simulink model "UAVFormation"  (R2021a)
settings: Solver=FixedStepAuto  StartTime=0.0  StopTime=150  FixedStep=0.1  RelTol=1e-3
(part 1 of 2)
settings Model: Creator=templ  LastModifiedBy=templ
settings DataIOCC: ReturnWorkspaceOutputs=off

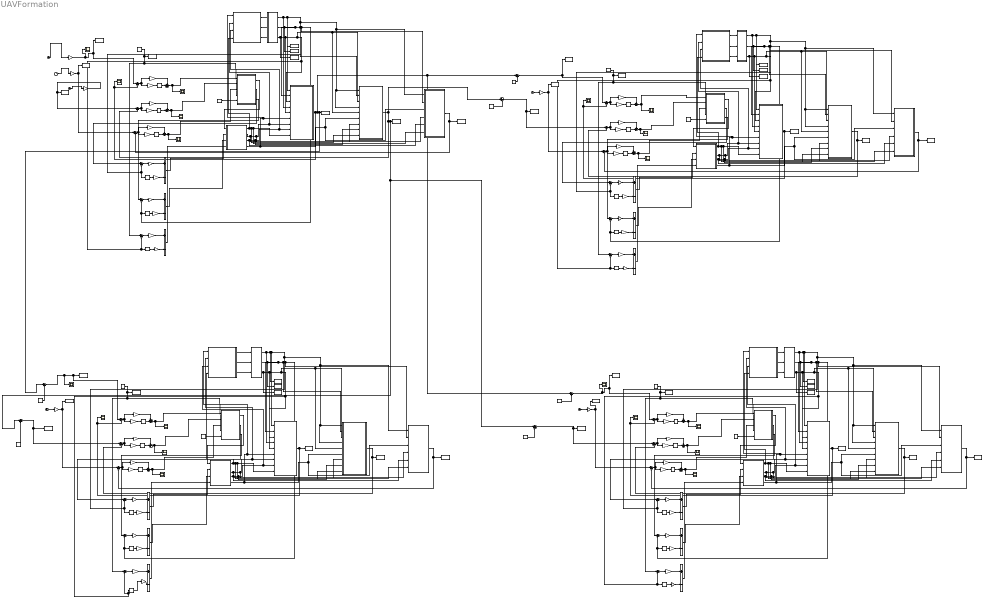
== system UAVFormation ==
  note: Attitude
  note: Position
  note: Attitude
  note: Position
  note: Attitude
  note: Position
  note: Attitude
  note: Position
  Add{1..12} (12 alike) : Sum  Inputs=+-
  Attitude Control Module1 : Subsystem
  Attitude Control Module2 : Subsystem
  Attitude Control Module3 : Subsystem
  Attitude Control Module4 : Subsystem
  Clock{,1,3,5,8,11} (6 alike) : Clock
  Constant{,1..5} (6 alike) : Constant  Value=5
  Derivative{1..24} (24 alike) : Derivative
  Gain{10,32,35,55} (4 alike) : Gain  Gain=0.05
  Gain{11,36,41,56} (4 alike) : Gain  Gain=0.32
  Gain{12..13,16,18,38,40,43,45,58,60} (10 alike) : Gain  Gain=0.2
  Gain{7,14,17,27,31,37,39,42,44,52,57,59} (12 alike) : Gain  Gain=0.5
  Gain{3,15,23,48} (4 alike) : Gain  Gain=0.1
  Gain{4,8,20,24,28,33,49,53} (8 alike) : Gain  Gain=0.6
  Gain{5,9,21,25,29,34,50,54} (8 alike) : Gain  Gain=0.8
  Gain{6,26,30,51} (4 alike) : Gain  Gain=0.25
  MATLAB Function1 : MATLAB Function  TreatAsAtomicUnit=on
  MATLAB Function2 : MATLAB Function  TreatAsAtomicUnit=on
  MATLAB Function3 : MATLAB Function  TreatAsAtomicUnit=on
  MATLAB Function4 : MATLAB Function  TreatAsAtomicUnit=on
  MATLAB Function5 : MATLAB Function  TreatAsAtomicUnit=on
  MATLAB Function6 : MATLAB Function  TreatAsAtomicUnit=on
  MATLAB Function7 : MATLAB Function  TreatAsAtomicUnit=on
  MATLAB Function8 : MATLAB Function  TreatAsAtomicUnit=on
  Position1 : MATLAB Function  TreatAsAtomicUnit=on
  Position2 : MATLAB Function  TreatAsAtomicUnit=on
  Position3 : MATLAB Function  TreatAsAtomicUnit=on
  Position4 : MATLAB Function  TreatAsAtomicUnit=on
  Scope{1..5,7..20} (19 alike) : Scope
  Subsystem1 : Subsystem
  Subsystem2 : Subsystem
  Subsystem3 : Subsystem
  Subsystem4 : Subsystem
  Subsystem5 : Subsystem
  Subsystem6 : Subsystem
  Subsystem7 : Subsystem
  Subsystem8 : Subsystem
  Sum{,2,4,6..9,11,13,15..18,21,23,25..28,30..31,33..38,41} (28 alike) : Sum  Inputs=|+-
  Sum{1,3,5,10,12,14,19..20,22,24,29,32} (12 alike) : Sum  Inputs=++|
  Sum39 : Sum  Inputs=|++
  Sum40 : Sum  Inputs=|++
  To Workspace1 : ToWorkspace  VariableName=theta1  SampleTime=-1
  To Workspace10 : ToWorkspace  VariableName=phi1  SampleTime=-1
  To Workspace11 : ToWorkspace  VariableName=xd1  SampleTime=-1
  To Workspace12 : ToWorkspace  VariableName=yd1  SampleTime=-1
  To Workspace13 : ToWorkspace  VariableName=zd1  SampleTime=-1
  To Workspace14 : ToWorkspace  VariableName=theta2  SampleTime=-1
  To Workspace15 : ToWorkspace  VariableName=psid2  SampleTime=-1
  To Workspace16 : ToWorkspace  VariableName=psi2  SampleTime=-1
  To Workspace17 : ToWorkspace  VariableName=x2  SampleTime=-1
  To Workspace18 : ToWorkspace  VariableName=y2  SampleTime=-1
  To Workspace19 : ToWorkspace  VariableName=z2  SampleTime=-1
  To Workspace2 : ToWorkspace  VariableName=psid1  SampleTime=-1
  To Workspace20 : ToWorkspace  VariableName=theta  SampleTime=-1
  To Workspace21 : ToWorkspace  VariableName=psid  SampleTime=-1
  To Workspace22 : ToWorkspace  VariableName=psi  SampleTime=-1
  To Workspace23 : ToWorkspace  VariableName=x  SampleTime=-1
  To Workspace24 : ToWorkspace  VariableName=y  SampleTime=-1
  To Workspace25 : ToWorkspace  VariableName=z  SampleTime=-1
  To Workspace26 : ToWorkspace  VariableName=phi2  SampleTime=-1
  To Workspace27 : ToWorkspace  VariableName=xd2  SampleTime=-1
  To Workspace28 : ToWorkspace  VariableName=yd2  SampleTime=-1
  To Workspace29 : ToWorkspace  VariableName=phi  SampleTime=-1
  To Workspace3 : ToWorkspace  VariableName=psi1  SampleTime=-1
  To Workspace30 : ToWorkspace  VariableName=zd2  SampleTime=-1
  To Workspace31 : ToWorkspace  VariableName=theta3  SampleTime=-1
  To Workspace32 : ToWorkspace  VariableName=psid3  SampleTime=-1
  To Workspace33 : ToWorkspace  VariableName=psi3  SampleTime=-1
  To Workspace34 : ToWorkspace  VariableName=x3  SampleTime=-1
  To Workspace35 : ToWorkspace  VariableName=y3  SampleTime=-1
  To Workspace36 : ToWorkspace  VariableName=z3  SampleTime=-1
  To Workspace37 : ToWorkspace  VariableName=phi3  SampleTime=-1
  To Workspace38 : ToWorkspace  VariableName=xd3  SampleTime=-1
  To Workspace39 : ToWorkspace  VariableName=yd3  SampleTime=-1
  To Workspace4 : ToWorkspace  VariableName=x1  SampleTime=-1
  To Workspace40 : ToWorkspace  VariableName=zd3  SampleTime=-1
  To Workspace5 : ToWorkspace  VariableName=y1  SampleTime=-1
  To Workspace6 : ToWorkspace  VariableName=xd  SampleTime=-1
  To Workspace7 : ToWorkspace  VariableName=yd  SampleTime=-1
  To Workspace8 : ToWorkspace  VariableName=zd  SampleTime=-1
  To Workspace9 : ToWorkspace  VariableName=z1  SampleTime=-1
  m{1..4} (4 alike) : Constant  Value=1.5
  psaid{1..4} (4 alike) : Constant  Value=0.2
  x1 : Subsystem
  x2 : Subsystem
  x3 : Subsystem
  x4 : Subsystem
  wires:
  MATLAB Function1/2(w2) -> Subsystem5/4(w2), Subsystem4/7(w2), Attitude Control Module2/2(w2), x2/7(w2)
  MATLAB Function1/3(w3) -> Subsystem5/5(w3), Subsystem4/8(w3), Attitude Control Module2/3(w3), x2/8(w3)
  MATLAB Function1/1(w1) -> Attitude Control Module2/4(w1), Subsystem4/9(w1), Subsystem5/6(w1), x2/9(w1)
  MATLAB Function1/4(w4) -> Subsystem5/3(w4), Subsystem4/6(w4), Attitude Control Module2/1(w4), x2/6(w4)
  Attitude Control Module2/1(phi) -> MATLAB Function5/1(u1)
  Attitude Control Module2/2(theta) -> MATLAB Function5/2(u2)
  Attitude Control Module2/3(psai) -> MATLAB Function5/3(u3)
  Gain20/1 -> Sum20/1
  Derivative16/1 -> Sum24/2
  Gain21/1 -> Derivative14/1
  Gain36/1 -> Derivative16/1
  Gain33/1 -> Sum22/1
  Sum30/1 -> Gain21/1, Gain20/1
  Derivative15/1 -> Sum22/2
  Sum21/1 -> Gain34/1, Gain33/1
  Subsystem5/1(Out1) -> Sum23/2, To Workspace25/1
  Gain35/1 -> Sum24/1
  Derivative14/1 -> Sum20/2
  Gain15/1 -> Sum23/1, To Workspace8/1
  Sum23/1 -> Gain36/1, Gain35/1
  Gain34/1 -> Derivative15/1
  Gain13/1 -> Sum21/1, To Workspace7/1
  Gain12/1 -> Scope3/1, To Workspace6/1, Sum30/1
  Position1/1(U1) -> MATLAB Function1/1(U1)
  Sum22/1 -> Scope12/1, Position1/2(Uy)
  Add8/1 -> MATLAB Function1/4(U4)
  m1/1 -> Position1/5(m)
  Add6/1 -> MATLAB Function1/2(U2)
  Sum24/1 -> Scope13/1, Position1/3(Uz)
  Add7/1 -> MATLAB Function1/3(U3)
  Sum20/1 -> Scope11/1, Position1/1(Ux)
  Sum27/1 -> Gain30/1
  Derivative13/1 -> Gain31/1
  Derivative17/1 -> Gain38/1
  Gain31/1 -> Add8/2
  Gain38/1 -> Add6/2
  Gain40/1 -> Add7/2
  MATLAB Function5/3(psai) -> To Workspace22/1, Subsystem4/5(In5), Subsystem4/3(psai), Sum27/2, Derivative13/1, x2/3(psai), x2/5(In5)
  Gain39/1 -> Add7/1
  Gain37/1 -> Add6/1
  Sum25/1 -> Gain37/1
  Position1/2(phid) -> Sum25/1
  Position1/3(thetad) -> Sum26/1
  Derivative12/1 -> Gain40/1
  psaid3/1 -> Sum27/1, Position1/4(psaid), To Workspace21/1
  Gain30/1 -> Add8/1
  MATLAB Function5/1(phi) -> x2/4(In4), To Workspace29/1, Derivative17/1, Sum25/2, Subsystem5/1(phi), Subsystem4/4(In4), Subsystem4/1(phi), x2/1(phi)
  MATLAB Function5/2(theta) -> To Workspace20/1, Sum26/2, Derivative12/1, Subsystem5/2(theta), Subsystem4/2(theta), x2/2(theta)
  Sum26/1 -> Gain39/1
  MATLAB Function2/4(w4) -> Subsystem2/3(w4), Subsystem1/6(w4), Attitude Control Module1/1(w4), x1/6(w4)
  Add1/1 -> MATLAB Function2/2(U2)
  Sum7/1 -> Gain17/1
  Sum37/1 -> Sum2/1, To Workspace12/1
  Clock5/1 -> Gain3/1
  Sum/1 -> To Workspace11/1, Sum9/1
  Gain6/1 -> Add3/1
  Sum6/1 -> Gain14/1
  Derivative1/1 -> Gain18/1
  Gain17/1 -> Add2/1
  Gain18/1 -> Add2/2
  Add2/1 -> MATLAB Function2/3(U3)
  Gain14/1 -> Add1/1
  Add3/1 -> MATLAB Function2/4(U4)
  Gain16/1 -> Add1/2
  Derivative2/1 -> Gain7/1
  Sum8/1 -> Gain6/1
  Derivative6/1 -> Gain16/1
  Gain3/1 -> Sum4/1, To Workspace13/1
  MATLAB Function2/1(w1) -> Attitude Control Module1/4(w1), Subsystem1/9(w1), Subsystem2/6(w1), x1/9(w1)
  m2/1 -> Position2/5(m)
  MATLAB Function2/3(w3) -> Subsystem2/5(w3), Subsystem1/8(w3), Attitude Control Module1/3(w3), x1/8(w3)
  Subsystem2/1(Out1) -> Sum4/2, To Workspace9/1
  x1/1(Out1) -> Sum9/2, Scope5/1, To Workspace4/1
  Gain9/1 -> Derivative4/1
  Sum1/1 -> Scope1/1, Position2/1(Ux)
  Position2/1(U1) -> MATLAB Function2/1(U1)
  Position2/2(phid) -> Sum6/1
  Gain4/1 -> Sum1/1
  Gain7/1 -> Add3/2
  Gain10/1 -> Sum5/1
  Sum2/1 -> Gain9/1, Gain8/1
  Derivative3/1 -> Sum1/2
  MATLAB Function2/2(w2) -> Subsystem2/4(w2), Subsystem1/7(w2), Attitude Control Module1/2(w2), x1/7(w2)
  MATLAB Function3/1(phi) -> x1/4(In4), To Workspace10/1, Derivative6/1, Sum6/2, Subsystem2/1(phi), Subsystem1/4(In4), Subsystem1/1(phi), x1/1(phi)
  Attitude Control Module1/3(psai) -> MATLAB Function3/3(u3)
  Sum5/1 -> Scope4/1, Position2/3(Uz)
  Position2/3(thetad) -> Sum7/1
  Sum4/1 -> Gain11/1, Gain10/1
  Gain8/1 -> Sum3/1
  Sum9/1 -> Gain5/1, Gain4/1
  Gain11/1 -> Derivative5/1
  Derivative5/1 -> Sum5/2
  Derivative4/1 -> Sum3/2
  Subsystem1/1(Out1) -> Sum2/2, To Workspace5/1
  Gain5/1 -> Derivative3/1
  Attitude Control Module1/2(theta) -> MATLAB Function3/2(u2)
  MATLAB Function3/3(psai) -> To Workspace3/1, Subsystem1/5(In5), Subsystem1/3(psai), Sum8/2, Derivative2/1, x1/3(psai), x1/5(In5)
  Sum3/1 -> Scope2/1, Position2/2(Uy)
  MATLAB Function3/2(theta) -> To Workspace1/1, Sum7/2, Derivative1/1, Subsystem2/2(theta), Subsystem1/2(theta), x1/2(theta)
  psaid1/1 -> Sum8/1, Position2/4(psaid), To Workspace2/1
  Attitude Control Module1/1(phi) -> MATLAB Function3/1(u1)
  MATLAB Function4/4(w4) -> Subsystem6/3(w4), Subsystem3/6(w4), Attitude Control Module3/1(w4), x3/6(w4)
  Add4/1 -> MATLAB Function4/2(U2)
  Sum16/1 -> Gain44/1
  Clock8/1 -> Gain23/1
  Gain26/1 -> Add9/1
  Sum15/1 -> Gain42/1
  Derivative7/1 -> Gain45/1
  Gain44/1 -> Add5/1
  Gain45/1 -> Add5/2
  Add5/1 -> MATLAB Function4/3(U3)
  Gain42/1 -> Add4/1
  Add9/1 -> MATLAB Function4/4(U4)
  Gain43/1 -> Add4/2
  Derivative8/1 -> Gain27/1
  Sum17/1 -> Gain26/1
  Derivative18/1 -> Gain43/1
  Gain23/1 -> Sum13/1, To Workspace30/1
  MATLAB Function4/1(w1) -> Attitude Control Module3/4(w1), Subsystem3/9(w1), Subsystem6/6(w1), x3/9(w1)
  m3/1 -> Position3/5(m)
  MATLAB Function4/3(w3) -> Subsystem6/5(w3), Subsystem3/8(w3), Attitude Control Module3/3(w3), x3/8(w3)
  Subsystem6/1(Out1) -> Sum13/2, To Workspace19/1
  x3/1(Out1) -> Sum18/2, Scope10/1, To Workspace17/1
  Gain29/1 -> Derivative10/1
  Sum10/1 -> Scope7/1, Position3/1(Ux)
  Position3/1(U1) -> MATLAB Function4/1(U1)
  Position3/2(phid) -> Sum15/1
  Gain24/1 -> Sum10/1
  Gain27/1 -> Add9/2
  Gain32/1 -> Sum14/1
  Sum11/1 -> Gain29/1, Gain28/1
  Derivative9/1 -> Sum10/2
  MATLAB Function4/2(w2) -> Subsystem6/4(w2), Subsystem3/7(w2), Attitude Control Module3/2(w2), x3/7(w2)
  MATLAB Function6/1(phi) -> x3/4(In4), To Workspace26/1, Derivative18/1, Sum15/2, Subsystem6/1(phi), Subsystem3/4(In4), Subsystem3/1(phi), x3/1(phi)
  Attitude Control Module3/3(psai) -> MATLAB Function6/3(u3)
  Sum14/1 -> Scope9/1, Position3/3(Uz)
  Position3/3(thetad) -> Sum16/1
  Sum13/1 -> Gain41/1, Gain32/1
  Gain28/1 -> Sum12/1
  Sum18/1 -> Gain25/1, Gain24/1
  Gain41/1 -> Derivative11/1
  Derivative11/1 -> Sum14/2
  Derivative10/1 -> Sum12/2
  Subsystem3/1(Out1) -> Sum11/2, To Workspace18/1
  Gain25/1 -> Derivative9/1
  Attitude Control Module3/2(theta) -> MATLAB Function6/2(u2)
  MATLAB Function6/3(psai) -> To Workspace16/1, Subsystem3/5(In5), Subsystem3/3(psai), Derivative8/1, Sum17/2, x3/3(psai), x3/5(In5)
  Sum12/1 -> Scope8/1, Position3/2(Uy)
  MATLAB Function6/2(theta) -> To Workspace14/1, Sum16/2, Derivative7/1, Subsystem6/2(theta), Subsystem3/2(theta), x3/2(theta)
  psaid2/1 -> Sum17/1, Position3/4(psaid), To Workspace15/1
  Attitude Control Module3/1(phi) -> MATLAB Function6/1(u1)
  MATLAB Function7/4(w4) -> Subsystem8/3(w4), Subsystem7/6(w4), Attitude Control Module4/1(w4), x4/6(w4)
  Add10/1 -> MATLAB Function7/2(U2)
  Sum34/1 -> Gain59/1
  Sum41/1 -> Sum28/1, To Workspace39/1
  Clock11/1 -> Gain48/1
  Sum40/1 -> Scope20/1, To Workspace38/1, Sum36/1
  Gain51/1 -> Add12/1
  Sum33/1 -> Gain57/1
  Derivative19/1 -> Gain60/1
  Gain59/1 -> Add11/1
  Gain60/1 -> Add11/2
  Add11/1 -> MATLAB Function7/3(U3)
  Gain57/1 -> Add10/1
  Add12/1 -> MATLAB Function7/4(U4)
  Gain58/1 -> Add10/2
  Derivative20/1 -> Gain52/1
  Sum35/1 -> Gain51/1
  Derivative24/1 -> Gain58/1
  Gain48/1 -> Sum31/1, To Workspace40/1
  MATLAB Function7/1(w1) -> Attitude Control Module4/4(w1), Subsystem7/9(w1), Subsystem8/6(w1), x4/9(w1)
  m4/1 -> Position4/5(m)
  MATLAB Function7/3(w3) -> Subsystem8/5(w3), Subsystem7/8(w3), Attitude Control Module4/3(w3), x4/8(w3)
  Subsystem8/1(Out1) -> Sum31/2, To Workspace36/1
  x4/1(Out1) -> Sum36/2, Scope19/1, To Workspace34/1
  Gain54/1 -> Derivative22/1
  Sum19/1 -> Scope16/1, Position4/1(Ux)
  Position4/1(U1) -> MATLAB Function7/1(U1)
  Position4/2(phid) -> Sum33/1
  Gain49/1 -> Sum19/1
  Gain52/1 -> Add12/2
  Gain55/1 -> Sum32/1
  Sum28/1 -> Gain54/1, Gain53/1
  Derivative21/1 -> Sum19/2
  MATLAB Function7/2(w2) -> Subsystem8/4(w2), Subsystem7/7(w2), Attitude Control Module4/2(w2), x4/7(w2)
  MATLAB Function8/1(phi) -> x4/4(In4), To Workspace37/1, Derivative24/1, Sum33/2, Subsystem8/1(phi), Subsystem7/4(In4), Subsystem7/1(phi), x4/1(phi)
  Attitude Control Module4/3(psai) -> MATLAB Function8/3(u3)
  Sum32/1 -> Scope18/1, Position4/3(Uz)
  Position4/3(thetad) -> Sum34/1
  Sum31/1 -> Gain56/1, Gain55/1
  Gain53/1 -> Sum29/1
  Sum36/1 -> Gain50/1, Gain49/1
  Gain56/1 -> Derivative23/1
  Derivative23/1 -> Sum32/2
  Derivative22/1 -> Sum29/2
  Subsystem7/1(Out1) -> Sum28/2, To Workspace35/1
  Gain50/1 -> Derivative21/1
  Attitude Control Module4/2(theta) -> MATLAB Function8/2(u2)
  MATLAB Function8/3(psai) -> To Workspace33/1, Subsystem7/5(In5), Subsystem7/3(psai), Sum35/2, Derivative20/1, x4/3(psai), x4/5(In5)
  Sum29/1 -> Scope17/1, Position4/2(Uy)
  MATLAB Function8/2(theta) -> To Workspace31/1, Sum34/2, Derivative19/1, Subsystem8/2(theta), Subsystem7/2(theta), x4/2(theta)
  psaid4/1 -> Sum35/1, Position4/4(psaid), To Workspace32/1
  Attitude Control Module4/1(phi) -> MATLAB Function8/1(u1)
  Constant/1 -> Sum/2
  Constant1/1 -> Sum37/2
  Constant2/1 -> Sum38/2
  Sum38/1 -> Scope15/1, Sum18/1, To Workspace27/1
  Sum39/1 -> Sum11/1, To Workspace28/1
  Constant3/1 -> Sum39/2
  Constant4/1 -> Sum40/2
  Constant5/1 -> Sum41/2
  x2/1(Out1) -> Sum30/2, Scope14/1, Sum40/1, Sum/1, Sum38/1, To Workspace23/1
  Subsystem4/1(Out1) -> Sum21/2, To Workspace24/1, Sum41/1, Sum39/1, Sum37/1
  Clock3/1 -> Gain15/1
  Clock/1 -> Gain12/1
  Clock1/1 -> Gain13/1

== system UAVFormation/Attitude Control Module1 ==
  note: phi
  note: theta
  note: psi
  w4 : Inport
  w2 : Inport  Port=2
  w3 : Inport  Port=3
  w1 : Inport  Port=4
  Integrator{,1..5} (6 alike) : Integrator
  Subsystem : Subsystem
  Subsystem1 : Subsystem
  Subsystem2 : Subsystem
  phi : Outport  VectorParamsAs1DForOutWhenUnconnected=off
  theta : Outport  Port=2  VectorParamsAs1DForOutWhenUnconnected=off
  psai : Outport  Port=3  VectorParamsAs1DForOutWhenUnconnected=off
  wires:
  w2/1 -> Subsystem2/2(w2), Subsystem/1(w2)
  Subsystem/1(Out1) -> Integrator1/1
  Integrator3/1 -> Subsystem2/4(In4), Subsystem/3(In3), Integrator2/1
  Integrator1/1 -> Subsystem2/3(In3), Subsystem1/3(In3), Integrator/1
  Integrator5/1 -> Subsystem/4(In4), Subsystem1/4(In4), Integrator4/1
  w4/1 -> Subsystem2/6(w4), Subsystem/2(w4)
  Subsystem2/1(Out1) -> Integrator5/1
  w1/1 -> Subsystem2/1(w1), Subsystem1/2(w1)
  Integrator2/1 -> theta/1
  Integrator/1 -> phi/1
  Integrator4/1 -> psai/1
  Subsystem1/1(Out1) -> Integrator3/1
  w3/1 -> Subsystem2/5(w3), Subsystem1/1(w3)

== system UAVFormation/Attitude Control Module2 ==
  note: phi
  note: theta
  note: psi
  w4 : Inport
  w2 : Inport  Port=2
  w3 : Inport  Port=3
  w1 : Inport  Port=4
  Integrator{,1..5} (6 alike) : Integrator
  Subsystem : Subsystem
  Subsystem1 : Subsystem
  Subsystem2 : Subsystem
  phi : Outport  VectorParamsAs1DForOutWhenUnconnected=off
  theta : Outport  Port=2  VectorParamsAs1DForOutWhenUnconnected=off
  psai : Outport  Port=3  VectorParamsAs1DForOutWhenUnconnected=off
  wires:
  w2/1 -> Subsystem2/2(w2), Subsystem/1(w2)
  Subsystem/1(Out1) -> Integrator1/1
  Integrator3/1 -> Subsystem2/4(In4), Subsystem/3(In3), Integrator2/1
  Integrator1/1 -> Subsystem2/3(In3), Subsystem1/3(In3), Integrator/1
  Integrator5/1 -> Subsystem/4(In4), Subsystem1/4(In4), Integrator4/1
  w4/1 -> Subsystem2/6(w4), Subsystem/2(w4)
  Subsystem2/1(Out1) -> Integrator5/1
  w1/1 -> Subsystem2/1(w1), Subsystem1/2(w1)
  Integrator2/1 -> theta/1
  Integrator/1 -> phi/1
  Integrator4/1 -> psai/1
  Subsystem1/1(Out1) -> Integrator3/1
  w3/1 -> Subsystem2/5(w3), Subsystem1/1(w3)

== system UAVFormation/Attitude Control Module3 ==
  note: phi
  note: theta
  note: psi
  w4 : Inport
  w2 : Inport  Port=2
  w3 : Inport  Port=3
  w1 : Inport  Port=4
  Integrator{,1..5} (6 alike) : Integrator
  Subsystem : Subsystem
  Subsystem1 : Subsystem
  Subsystem2 : Subsystem
  phi : Outport  VectorParamsAs1DForOutWhenUnconnected=off
  theta : Outport  Port=2  VectorParamsAs1DForOutWhenUnconnected=off
  psai : Outport  Port=3  VectorParamsAs1DForOutWhenUnconnected=off
  wires:
  w2/1 -> Subsystem2/2(w2), Subsystem/1(w2)
  Subsystem/1(Out1) -> Integrator1/1
  Integrator3/1 -> Subsystem2/4(In4), Subsystem/3(In3), Integrator2/1
  Integrator1/1 -> Subsystem2/3(In3), Subsystem1/3(In3), Integrator/1
  Integrator5/1 -> Subsystem/4(In4), Subsystem1/4(In4), Integrator4/1
  w4/1 -> Subsystem2/6(w4), Subsystem/2(w4)
  Subsystem2/1(Out1) -> Integrator5/1
  w1/1 -> Subsystem2/1(w1), Subsystem1/2(w1)
  Integrator2/1 -> theta/1
  Integrator/1 -> phi/1
  Integrator4/1 -> psai/1
  Subsystem1/1(Out1) -> Integrator3/1
  w3/1 -> Subsystem2/5(w3), Subsystem1/1(w3)

== system UAVFormation/Attitude Control Module4 ==
  note: phi
  note: theta
  note: psi
  w4 : Inport
  w2 : Inport  Port=2
  w3 : Inport  Port=3
  w1 : Inport  Port=4
  Integrator{,1..5} (6 alike) : Integrator
  Subsystem : Subsystem
  Subsystem1 : Subsystem
  Subsystem2 : Subsystem
  phi : Outport  VectorParamsAs1DForOutWhenUnconnected=off
  theta : Outport  Port=2  VectorParamsAs1DForOutWhenUnconnected=off
  psai : Outport  Port=3  VectorParamsAs1DForOutWhenUnconnected=off
  wires:
  w2/1 -> Subsystem2/2(w2), Subsystem/1(w2)
  Subsystem/1(Out1) -> Integrator1/1
  Integrator3/1 -> Subsystem2/4(In4), Subsystem/3(In3), Integrator2/1
  Integrator1/1 -> Subsystem2/3(In3), Subsystem1/3(In3), Integrator/1
  Integrator5/1 -> Subsystem/4(In4), Subsystem1/4(In4), Integrator4/1
  w4/1 -> Subsystem2/6(w4), Subsystem/2(w4)
  Subsystem2/1(Out1) -> Integrator5/1
  w1/1 -> Subsystem2/1(w1), Subsystem1/2(w1)
  Integrator2/1 -> theta/1
  Integrator/1 -> phi/1
  Integrator4/1 -> psai/1
  Subsystem1/1(Out1) -> Integrator3/1
  w3/1 -> Subsystem2/5(w3), Subsystem1/1(w3)

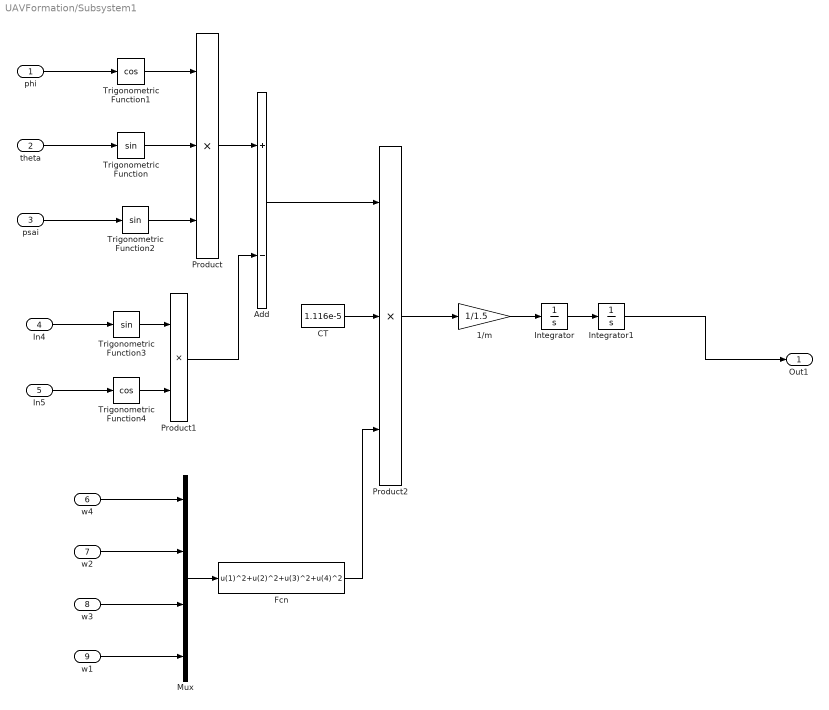
== system UAVFormation/Subsystem1 ==
  phi : Inport
  theta : Inport  Port=2
  psai : Inport  Port=3
  In4 : Inport  Port=4
  In5 : Inport  Port=5
  w4 : Inport  Port=6
  w2 : Inport  Port=7
  w3 : Inport  Port=8
  w1 : Inport  Port=9
  1/m : Gain  Gain=1/1.5
  Add : Sum  Inputs=+-
  CT : Constant  Value=1.116e-5
  Fcn : Fcn  Expr=u(1)^2+u(2)^2+u(3)^2+u(4)^2
  Integrator : Integrator
  Integrator1 : Integrator
  Mux : Mux
  Product : Product  Inputs=3
  Product1 : Product
  Product2 : Product  Inputs=3
  Trigonometric Function : Trigonometry
  Trigonometric Function1 : Trigonometry  Operator=cos
  Trigonometric Function2 : Trigonometry
  Trigonometric Function3 : Trigonometry
  Trigonometric Function4 : Trigonometry  Operator=cos
  Out1 : Outport  VectorParamsAs1DForOutWhenUnconnected=off
  wires:
  Mux/1 -> Fcn/1
  Product2/1 -> 1/m/1
  Fcn/1 -> Product2/3
  CT/1 -> Product2/2
  Trigonometric Function2/1 -> Product/3
  Trigonometric Function/1 -> Product/2
  Trigonometric Function3/1 -> Product1/1
  Product1/1 -> Add/2
  Product/1 -> Add/1
  Add/1 -> Product2/1
  In4/1 -> Trigonometric Function3/1
  Trigonometric Function1/1 -> Product/1
  Integrator/1 -> Integrator1/1
  w3/1 -> Mux/3
  Trigonometric Function4/1 -> Product1/2
  1/m/1 -> Integrator/1
  Integrator1/1 -> Out1/1
  w1/1 -> Mux/4
  phi/1 -> Trigonometric Function1/1
  w4/1 -> Mux/1
  In5/1 -> Trigonometric Function4/1
  w2/1 -> Mux/2
  psai/1 -> Trigonometric Function2/1
  theta/1 -> Trigonometric Function/1

== system UAVFormation/Subsystem2 ==
  phi : Inport
  theta : Inport  Port=2
  w4 : Inport  Port=3
  w2 : Inport  Port=4
  w3 : Inport  Port=5
  w1 : Inport  Port=6
  1/m : Gain  Gain=1/1.5
  Add : Sum  Inputs=+-
  CT : Constant  Value=1.116e-5
  Fcn : Fcn  Expr=u(1)^2+u(2)^2+u(3)^2+u(4)^2
  Integrator : Integrator
  Integrator1 : Integrator
  Mux : Mux
  Product1 : Product  Inputs=4
  Trigonometric Function : Trigonometry  Operator=cos
  Trigonometric Function1 : Trigonometry  Operator=cos
  mg : Constant  Value=1.5*9.81
  Out1 : Outport  VectorParamsAs1DForOutWhenUnconnected=off
  wires:
  Trigonometric Function1/1 -> Product1/1
  Integrator/1 -> Integrator1/1
  Fcn/1 -> Product1/4
  mg/1 -> Add/2
  CT/1 -> Product1/3
  Add/1 -> 1/m/1
  Mux/1 -> Fcn/1
  theta/1 -> Trigonometric Function/1
  1/m/1 -> Integrator/1
  Trigonometric Function/1 -> Product1/2
  Product1/1 -> Add/1
  w2/1 -> Mux/2
  Integrator1/1 -> Out1/1
  w3/1 -> Mux/3
  w4/1 -> Mux/1
  w1/1 -> Mux/4
  phi/1 -> Trigonometric Function1/1

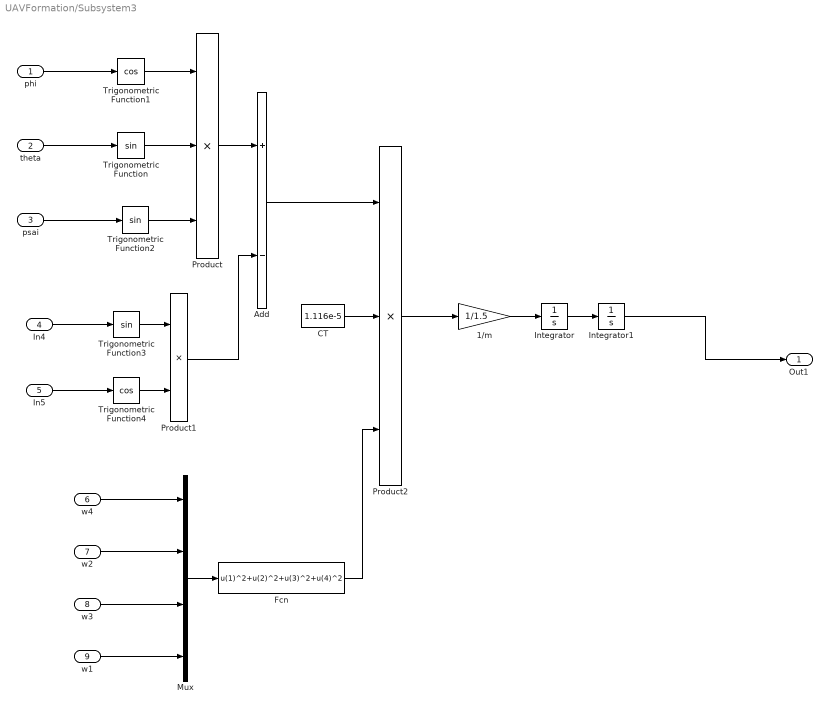
== system UAVFormation/Subsystem3 ==
  phi : Inport
  theta : Inport  Port=2
  psai : Inport  Port=3
  In4 : Inport  Port=4
  In5 : Inport  Port=5
  w4 : Inport  Port=6
  w2 : Inport  Port=7
  w3 : Inport  Port=8
  w1 : Inport  Port=9
  1/m : Gain  Gain=1/1.5
  Add : Sum  Inputs=+-
  CT : Constant  Value=1.116e-5
  Fcn : Fcn  Expr=u(1)^2+u(2)^2+u(3)^2+u(4)^2
  Integrator : Integrator
  Integrator1 : Integrator
  Mux : Mux
  Product : Product  Inputs=3
  Product1 : Product
  Product2 : Product  Inputs=3
  Trigonometric Function : Trigonometry
  Trigonometric Function1 : Trigonometry  Operator=cos
  Trigonometric Function2 : Trigonometry
  Trigonometric Function3 : Trigonometry
  Trigonometric Function4 : Trigonometry  Operator=cos
  Out1 : Outport  VectorParamsAs1DForOutWhenUnconnected=off
  wires:
  Mux/1 -> Fcn/1
  Product2/1 -> 1/m/1
  Fcn/1 -> Product2/3
  CT/1 -> Product2/2
  Trigonometric Function2/1 -> Product/3
  Trigonometric Function/1 -> Product/2
  Trigonometric Function3/1 -> Product1/1
  Product1/1 -> Add/2
  Product/1 -> Add/1
  Add/1 -> Product2/1
  In4/1 -> Trigonometric Function3/1
  Trigonometric Function1/1 -> Product/1
  Integrator/1 -> Integrator1/1
  w3/1 -> Mux/3
  Trigonometric Function4/1 -> Product1/2
  1/m/1 -> Integrator/1
  Integrator1/1 -> Out1/1
  w1/1 -> Mux/4
  phi/1 -> Trigonometric Function1/1
  w4/1 -> Mux/1
  In5/1 -> Trigonometric Function4/1
  w2/1 -> Mux/2
  psai/1 -> Trigonometric Function2/1
  theta/1 -> Trigonometric Function/1

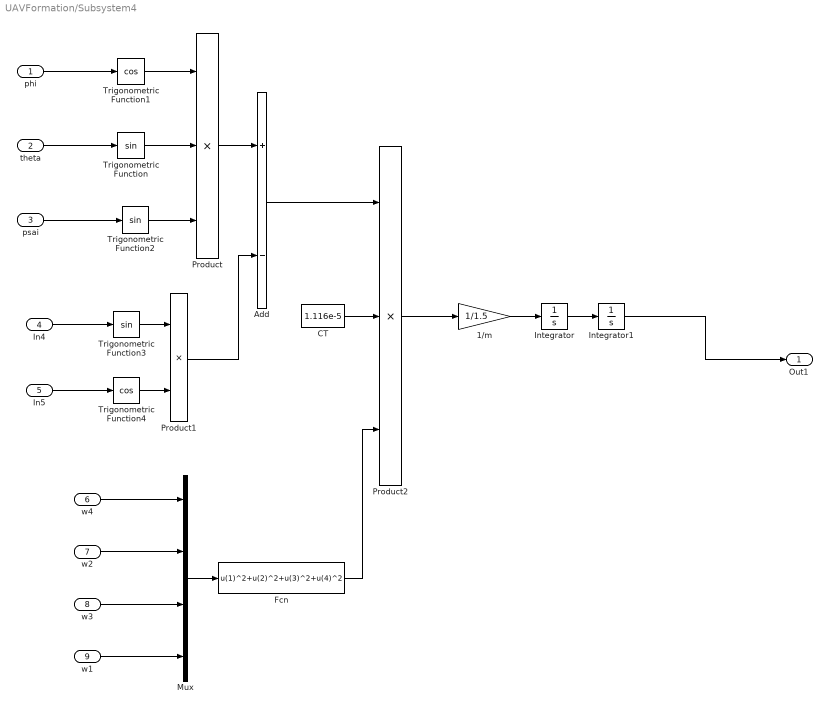
== system UAVFormation/Subsystem4 ==
  phi : Inport
  theta : Inport  Port=2
  psai : Inport  Port=3
  In4 : Inport  Port=4
  In5 : Inport  Port=5
  w4 : Inport  Port=6
  w2 : Inport  Port=7
  w3 : Inport  Port=8
  w1 : Inport  Port=9
  1/m : Gain  Gain=1/1.5
  Add : Sum  Inputs=+-
  CT : Constant  Value=1.116e-5
  Fcn : Fcn  Expr=u(1)^2+u(2)^2+u(3)^2+u(4)^2
  Integrator : Integrator
  Integrator1 : Integrator
  Mux : Mux
  Product : Product  Inputs=3
  Product1 : Product
  Product2 : Product  Inputs=3
  Trigonometric Function : Trigonometry
  Trigonometric Function1 : Trigonometry  Operator=cos
  Trigonometric Function2 : Trigonometry
  Trigonometric Function3 : Trigonometry
  Trigonometric Function4 : Trigonometry  Operator=cos
  Out1 : Outport  VectorParamsAs1DForOutWhenUnconnected=off
  wires:
  Mux/1 -> Fcn/1
  Product2/1 -> 1/m/1
  Fcn/1 -> Product2/3
  CT/1 -> Product2/2
  Trigonometric Function2/1 -> Product/3
  Trigonometric Function/1 -> Product/2
  Trigonometric Function3/1 -> Product1/1
  Product1/1 -> Add/2
  Product/1 -> Add/1
  Add/1 -> Product2/1
  In4/1 -> Trigonometric Function3/1
  Trigonometric Function1/1 -> Product/1
  Integrator/1 -> Integrator1/1
  w3/1 -> Mux/3
  Trigonometric Function4/1 -> Product1/2
  1/m/1 -> Integrator/1
  Integrator1/1 -> Out1/1
  w1/1 -> Mux/4
  phi/1 -> Trigonometric Function1/1
  w4/1 -> Mux/1
  In5/1 -> Trigonometric Function4/1
  w2/1 -> Mux/2
  psai/1 -> Trigonometric Function2/1
  theta/1 -> Trigonometric Function/1

== system UAVFormation/Subsystem5 ==
  phi : Inport
  theta : Inport  Port=2
  w4 : Inport  Port=3
  w2 : Inport  Port=4
  w3 : Inport  Port=5
  w1 : Inport  Port=6
  1/m : Gain  Gain=1/1.5
  Add : Sum  Inputs=+-
  CT : Constant  Value=1.116e-5
  Fcn : Fcn  Expr=u(1)^2+u(2)^2+u(3)^2+u(4)^2
  Integrator : Integrator
  Integrator1 : Integrator
  Mux : Mux
  Product1 : Product  Inputs=4
  Trigonometric Function : Trigonometry  Operator=cos
  Trigonometric Function1 : Trigonometry  Operator=cos
  mg : Constant  Value=1.5*9.81
  Out1 : Outport  VectorParamsAs1DForOutWhenUnconnected=off
  wires:
  Trigonometric Function1/1 -> Product1/1
  Integrator/1 -> Integrator1/1
  Fcn/1 -> Product1/4
  mg/1 -> Add/2
  CT/1 -> Product1/3
  Add/1 -> 1/m/1
  Mux/1 -> Fcn/1
  theta/1 -> Trigonometric Function/1
  1/m/1 -> Integrator/1
  Trigonometric Function/1 -> Product1/2
  Product1/1 -> Add/1
  w2/1 -> Mux/2
  Integrator1/1 -> Out1/1
  w3/1 -> Mux/3
  w4/1 -> Mux/1
  w1/1 -> Mux/4
  phi/1 -> Trigonometric Function1/1

== system UAVFormation/Subsystem6 ==
  phi : Inport
  theta : Inport  Port=2
  w4 : Inport  Port=3
  w2 : Inport  Port=4
  w3 : Inport  Port=5
  w1 : Inport  Port=6
  1/m : Gain  Gain=1/1.5
  Add : Sum  Inputs=+-
  CT : Constant  Value=1.116e-5
  Fcn : Fcn  Expr=u(1)^2+u(2)^2+u(3)^2+u(4)^2
  Integrator : Integrator
  Integrator1 : Integrator
  Mux : Mux
  Product1 : Product  Inputs=4
  Trigonometric Function : Trigonometry  Operator=cos
  Trigonometric Function1 : Trigonometry  Operator=cos
  mg : Constant  Value=1.5*9.81
  Out1 : Outport  VectorParamsAs1DForOutWhenUnconnected=off
  wires:
  Trigonometric Function1/1 -> Product1/1
  Integrator/1 -> Integrator1/1
  Fcn/1 -> Product1/4
  mg/1 -> Add/2
  CT/1 -> Product1/3
  Add/1 -> 1/m/1
  Mux/1 -> Fcn/1
  theta/1 -> Trigonometric Function/1
  1/m/1 -> Integrator/1
  Trigonometric Function/1 -> Product1/2
  Product1/1 -> Add/1
  w2/1 -> Mux/2
  Integrator1/1 -> Out1/1
  w3/1 -> Mux/3
  w4/1 -> Mux/1
  w1/1 -> Mux/4
  phi/1 -> Trigonometric Function1/1

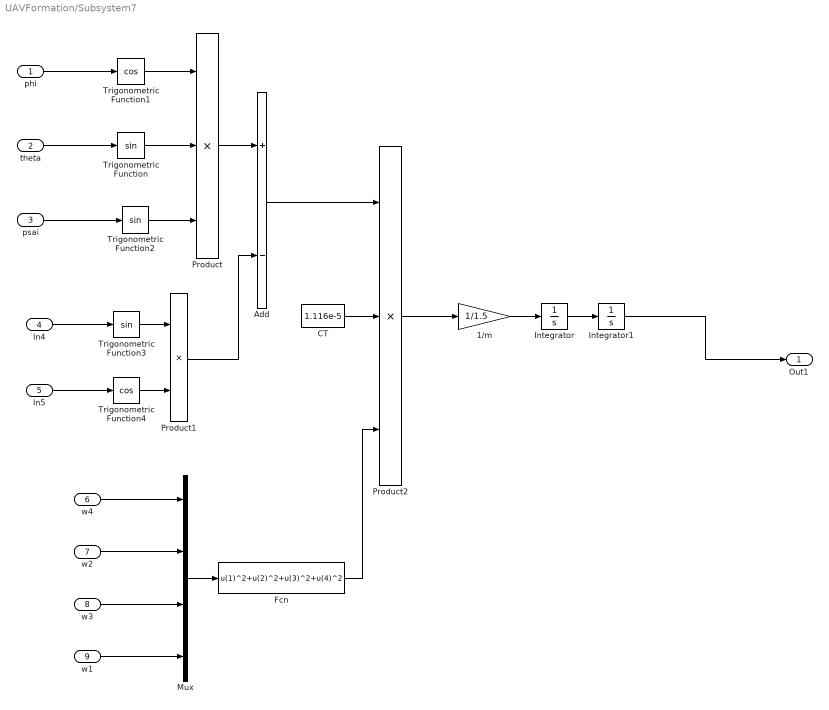
== system UAVFormation/Subsystem7 ==
  phi : Inport
  theta : Inport  Port=2
  psai : Inport  Port=3
  In4 : Inport  Port=4
  In5 : Inport  Port=5
  w4 : Inport  Port=6
  w2 : Inport  Port=7
  w3 : Inport  Port=8
  w1 : Inport  Port=9
  1/m : Gain  Gain=1/1.5
  Add : Sum  Inputs=+-
  CT : Constant  Value=1.116e-5
  Fcn : Fcn  Expr=u(1)^2+u(2)^2+u(3)^2+u(4)^2
  Integrator : Integrator
  Integrator1 : Integrator
  Mux : Mux
  Product : Product  Inputs=3
  Product1 : Product
  Product2 : Product  Inputs=3
  Trigonometric Function : Trigonometry
  Trigonometric Function1 : Trigonometry  Operator=cos
  Trigonometric Function2 : Trigonometry
  Trigonometric Function3 : Trigonometry
  Trigonometric Function4 : Trigonometry  Operator=cos
  Out1 : Outport  VectorParamsAs1DForOutWhenUnconnected=off
  wires:
  Mux/1 -> Fcn/1
  Product2/1 -> 1/m/1
  Fcn/1 -> Product2/3
  CT/1 -> Product2/2
  Trigonometric Function2/1 -> Product/3
  Trigonometric Function/1 -> Product/2
  Trigonometric Function3/1 -> Product1/1
  Product1/1 -> Add/2
  Product/1 -> Add/1
  Add/1 -> Product2/1
  In4/1 -> Trigonometric Function3/1
  Trigonometric Function1/1 -> Product/1
  Integrator/1 -> Integrator1/1
  w3/1 -> Mux/3
  Trigonometric Function4/1 -> Product1/2
  1/m/1 -> Integrator/1
  Integrator1/1 -> Out1/1
  w1/1 -> Mux/4
  phi/1 -> Trigonometric Function1/1
  w4/1 -> Mux/1
  In5/1 -> Trigonometric Function4/1
  w2/1 -> Mux/2
  psai/1 -> Trigonometric Function2/1
  theta/1 -> Trigonometric Function/1

== system UAVFormation/Subsystem8 ==
  phi : Inport
  theta : Inport  Port=2
  w4 : Inport  Port=3
  w2 : Inport  Port=4
  w3 : Inport  Port=5
  w1 : Inport  Port=6
  1/m : Gain  Gain=1/1.5
  Add : Sum  Inputs=+-
  CT : Constant  Value=1.116e-5
  Fcn : Fcn  Expr=u(1)^2+u(2)^2+u(3)^2+u(4)^2
  Integrator : Integrator
  Integrator1 : Integrator
  Mux : Mux
  Product1 : Product  Inputs=4
  Trigonometric Function : Trigonometry  Operator=cos
  Trigonometric Function1 : Trigonometry  Operator=cos
  mg : Constant  Value=1.5*9.81
  Out1 : Outport  VectorParamsAs1DForOutWhenUnconnected=off
  wires:
  Trigonometric Function1/1 -> Product1/1
  Integrator/1 -> Integrator1/1
  Fcn/1 -> Product1/4
  mg/1 -> Add/2
  CT/1 -> Product1/3
  Add/1 -> 1/m/1
  Mux/1 -> Fcn/1
  theta/1 -> Trigonometric Function/1
  1/m/1 -> Integrator/1
  Trigonometric Function/1 -> Product1/2
  Product1/1 -> Add/1
  w2/1 -> Mux/2
  Integrator1/1 -> Out1/1
  w3/1 -> Mux/3
  w4/1 -> Mux/1
  w1/1 -> Mux/4
  phi/1 -> Trigonometric Function1/1

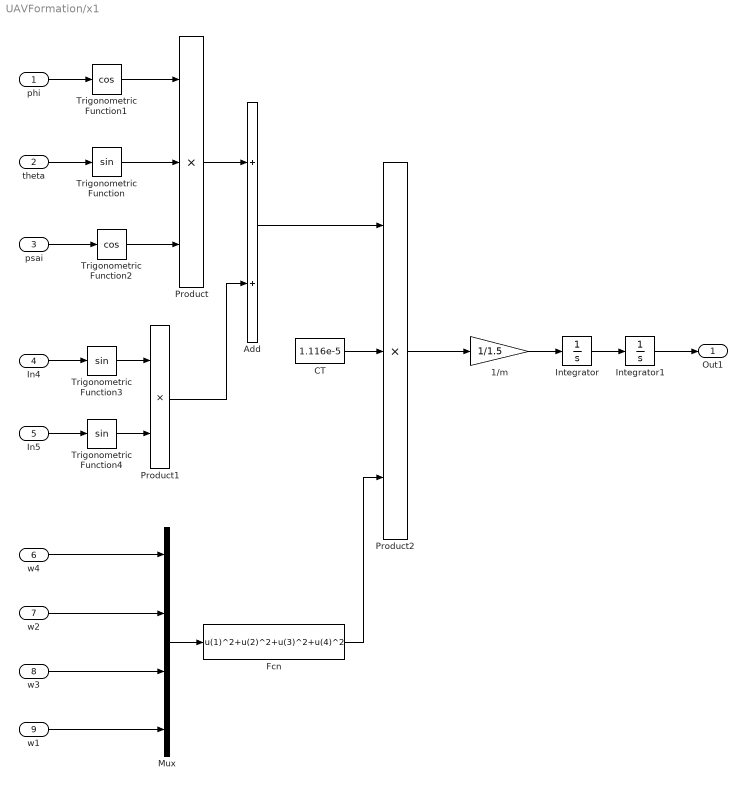
== system UAVFormation/x1 ==
  phi : Inport
  theta : Inport  Port=2
  psai : Inport  Port=3
  In4 : Inport  Port=4
  In5 : Inport  Port=5
  w4 : Inport  Port=6
  w2 : Inport  Port=7
  w3 : Inport  Port=8
  w1 : Inport  Port=9
  1/m : Gain  Gain=1/1.5
  Add : Sum
  CT : Constant  Value=1.116e-5
  Fcn : Fcn  Expr=u(1)^2+u(2)^2+u(3)^2+u(4)^2
  Integrator : Integrator
  Integrator1 : Integrator
  Mux : Mux
  Product : Product  Inputs=3
  Product1 : Product
  Product2 : Product  Inputs=3
  Trigonometric Function : Trigonometry
  Trigonometric Function1 : Trigonometry  Operator=cos
  Trigonometric Function2 : Trigonometry  Operator=cos
  Trigonometric Function3 : Trigonometry
  Trigonometric Function4 : Trigonometry
  Out1 : Outport  VectorParamsAs1DForOutWhenUnconnected=off
  wires:
  w3/1 -> Mux/3
  Integrator1/1 -> Out1/1
  1/m/1 -> Integrator/1
  Trigonometric Function4/1 -> Product1/2
  Integrator/1 -> Integrator1/1
  w2/1 -> Mux/2
  Add/1 -> Product2/1
  Product1/1 -> Add/2
  Product/1 -> Add/1
  In4/1 -> Trigonometric Function3/1
  Fcn/1 -> Product2/3
  Trigonometric Function1/1 -> Product/1
  theta/1 -> Trigonometric Function/1
  Trigonometric Function/1 -> Product/2
  Trigonometric Function2/1 -> Product/3
  Trigonometric Function3/1 -> Product1/1
  CT/1 -> Product2/2
  phi/1 -> Trigonometric Function1/1
  Product2/1 -> 1/m/1
  psai/1 -> Trigonometric Function2/1
  Mux/1 -> Fcn/1
  w4/1 -> Mux/1
  In5/1 -> Trigonometric Function4/1
  w1/1 -> Mux/4

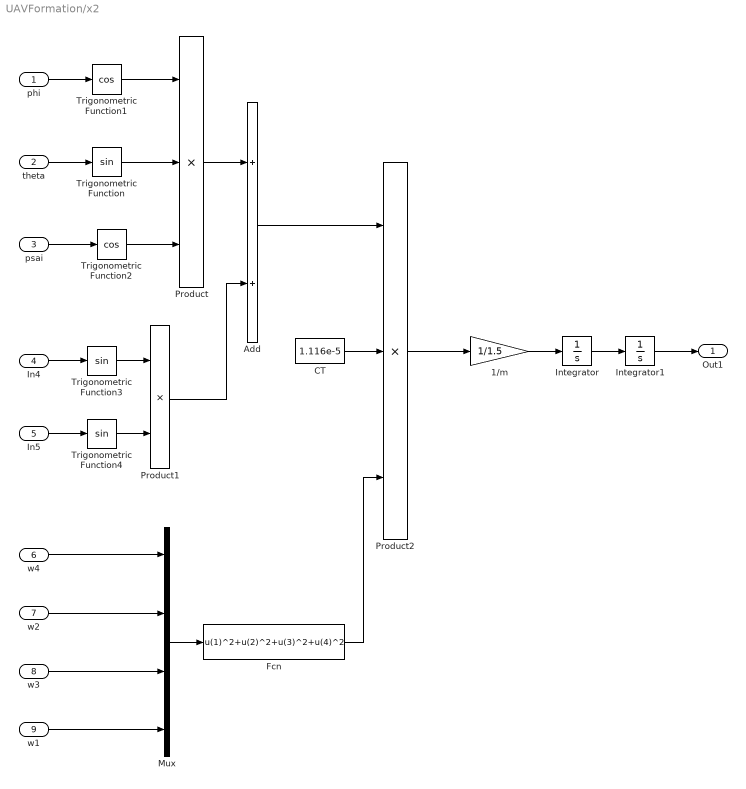
== system UAVFormation/x2 ==
  phi : Inport
  theta : Inport  Port=2
  psai : Inport  Port=3
  In4 : Inport  Port=4
  In5 : Inport  Port=5
  w4 : Inport  Port=6
  w2 : Inport  Port=7
  w3 : Inport  Port=8
  w1 : Inport  Port=9
  1/m : Gain  Gain=1/1.5
  Add : Sum
  CT : Constant  Value=1.116e-5
  Fcn : Fcn  Expr=u(1)^2+u(2)^2+u(3)^2+u(4)^2
  Integrator : Integrator
  Integrator1 : Integrator
  Mux : Mux
  Product : Product  Inputs=3
  Product1 : Product
  Product2 : Product  Inputs=3
  Trigonometric Function : Trigonometry
  Trigonometric Function1 : Trigonometry  Operator=cos
  Trigonometric Function2 : Trigonometry  Operator=cos
  Trigonometric Function3 : Trigonometry
  Trigonometric Function4 : Trigonometry
  Out1 : Outport  VectorParamsAs1DForOutWhenUnconnected=off
  wires:
  w3/1 -> Mux/3
  Integrator1/1 -> Out1/1
  1/m/1 -> Integrator/1
  Trigonometric Function4/1 -> Product1/2
  Integrator/1 -> Integrator1/1
  w2/1 -> Mux/2
  Add/1 -> Product2/1
  Product1/1 -> Add/2
  Product/1 -> Add/1
  In4/1 -> Trigonometric Function3/1
  Fcn/1 -> Product2/3
  Trigonometric Function1/1 -> Product/1
  theta/1 -> Trigonometric Function/1
  Trigonometric Function/1 -> Product/2
  Trigonometric Function2/1 -> Product/3
  Trigonometric Function3/1 -> Product1/1
  CT/1 -> Product2/2
  phi/1 -> Trigonometric Function1/1
  Product2/1 -> 1/m/1
  psai/1 -> Trigonometric Function2/1
  Mux/1 -> Fcn/1
  w4/1 -> Mux/1
  In5/1 -> Trigonometric Function4/1
  w1/1 -> Mux/4

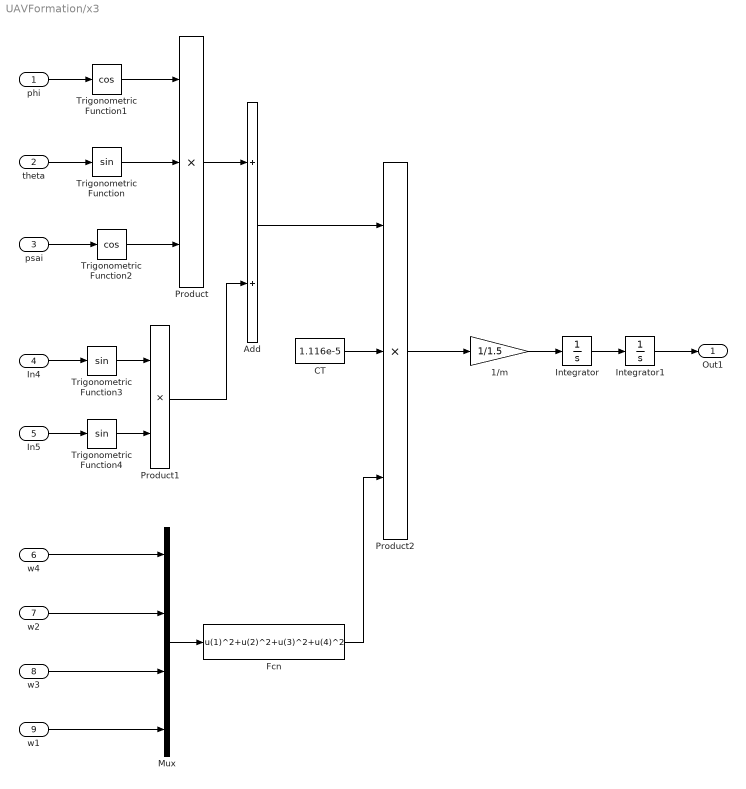
== system UAVFormation/x3 ==
  phi : Inport
  theta : Inport  Port=2
  psai : Inport  Port=3
  In4 : Inport  Port=4
  In5 : Inport  Port=5
  w4 : Inport  Port=6
  w2 : Inport  Port=7
  w3 : Inport  Port=8
  w1 : Inport  Port=9
  1/m : Gain  Gain=1/1.5
  Add : Sum
  CT : Constant  Value=1.116e-5
  Fcn : Fcn  Expr=u(1)^2+u(2)^2+u(3)^2+u(4)^2
  Integrator : Integrator
  Integrator1 : Integrator
  Mux : Mux
  Product : Product  Inputs=3
  Product1 : Product
  Product2 : Product  Inputs=3
  Trigonometric Function : Trigonometry
  Trigonometric Function1 : Trigonometry  Operator=cos
  Trigonometric Function2 : Trigonometry  Operator=cos
  Trigonometric Function3 : Trigonometry
  Trigonometric Function4 : Trigonometry
  Out1 : Outport  VectorParamsAs1DForOutWhenUnconnected=off
  wires:
  w3/1 -> Mux/3
  Integrator1/1 -> Out1/1
  1/m/1 -> Integrator/1
  Trigonometric Function4/1 -> Product1/2
  Integrator/1 -> Integrator1/1
  w2/1 -> Mux/2
  Add/1 -> Product2/1
  Product1/1 -> Add/2
  Product/1 -> Add/1
  In4/1 -> Trigonometric Function3/1
  Fcn/1 -> Product2/3
  Trigonometric Function1/1 -> Product/1
  theta/1 -> Trigonometric Function/1
  Trigonometric Function/1 -> Product/2
  Trigonometric Function2/1 -> Product/3
  Trigonometric Function3/1 -> Product1/1
  CT/1 -> Product2/2
  phi/1 -> Trigonometric Function1/1
  Product2/1 -> 1/m/1
  psai/1 -> Trigonometric Function2/1
  Mux/1 -> Fcn/1
  w4/1 -> Mux/1
  In5/1 -> Trigonometric Function4/1
  w1/1 -> Mux/4

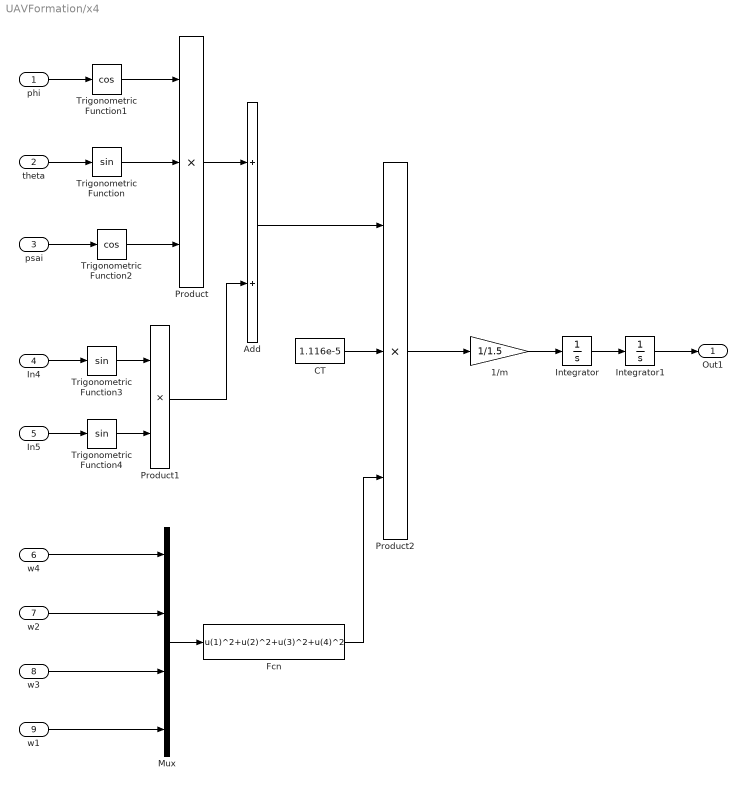
== system UAVFormation/x4 ==
  phi : Inport
  theta : Inport  Port=2
  psai : Inport  Port=3
  In4 : Inport  Port=4
  In5 : Inport  Port=5
  w4 : Inport  Port=6
  w2 : Inport  Port=7
  w3 : Inport  Port=8
  w1 : Inport  Port=9
  1/m : Gain  Gain=1/1.5
  Add : Sum
  CT : Constant  Value=1.116e-5
  Fcn : Fcn  Expr=u(1)^2+u(2)^2+u(3)^2+u(4)^2
  Integrator : Integrator
  Integrator1 : Integrator
  Mux : Mux
  Product : Product  Inputs=3
  Product1 : Product
  Product2 : Product  Inputs=3
  Trigonometric Function : Trigonometry
  Trigonometric Function1 : Trigonometry  Operator=cos
  Trigonometric Function2 : Trigonometry  Operator=cos
  Trigonometric Function3 : Trigonometry
  Trigonometric Function4 : Trigonometry
  Out1 : Outport  VectorParamsAs1DForOutWhenUnconnected=off
  wires:
  w3/1 -> Mux/3
  Integrator1/1 -> Out1/1
  1/m/1 -> Integrator/1
  Trigonometric Function4/1 -> Product1/2
  Integrator/1 -> Integrator1/1
  w2/1 -> Mux/2
  Add/1 -> Product2/1
  Product1/1 -> Add/2
  Product/1 -> Add/1
  In4/1 -> Trigonometric Function3/1
  Fcn/1 -> Product2/3
  Trigonometric Function1/1 -> Product/1
  theta/1 -> Trigonometric Function/1
  Trigonometric Function/1 -> Product/2
  Trigonometric Function2/1 -> Product/3
  Trigonometric Function3/1 -> Product1/1
  CT/1 -> Product2/2
  phi/1 -> Trigonometric Function1/1
  Product2/1 -> 1/m/1
  psai/1 -> Trigonometric Function2/1
  Mux/1 -> Fcn/1
  w4/1 -> Mux/1
  In5/1 -> Trigonometric Function4/1
  w1/1 -> Mux/4

== system UAVFormation/Attitude Control Module1/Subsystem ==
  w2 : Inport
  w4 : Inport  Port=2
  In3 : Inport  Port=3
  In4 : Inport  Port=4
  1/Jxx : Gain  Gain=1/(1.745e-2)
  Add : Sum  Inputs=+-
  Add1 : Sum
  Add2 : Sum  Inputs=+-
  CT : Constant  Value=1.116e-5
  Fcn : Fcn  Expr=u(1)^2
  Fcn1 : Fcn  Expr=u(1)^2
  Jyy : Constant  Value=1.745e-2
  "Jzz " : Constant  Value=3.175e-2
  Product : Product
  Product1 : Product
  Product2 : Product  Inputs=3
  d : Constant  Value=0.225
  Out1 : Outport  VectorParamsAs1DForOutWhenUnconnected=off
  wires:
  Product2/1 -> Add1/1
  Fcn/1 -> Add2/2
  CT/1 -> Product2/3
  "Jzz "/1 -> Add/2
  Add1/1 -> 1/Jxx/1
  Fcn1/1 -> Add2/1
  Add2/1 -> Product2/1
  Product1/1 -> Add1/2
  Product/1 -> Product1/2
  d/1 -> Product2/2
  In4/1 -> Product/2
  Jyy/1 -> Add/1
  w4/1 -> Fcn/1
  Add/1 -> Product1/1
  1/Jxx/1 -> Out1/1
  w2/1 -> Fcn1/1
  In3/1 -> Product/1

== system UAVFormation/Attitude Control Module1/Subsystem1 ==
  w3 : Inport
  w1 : Inport  Port=2
  In3 : Inport  Port=3
  In4 : Inport  Port=4
  1/Jxx : Gain  Gain=1/(1.745e-2)
  Add : Sum  Inputs=+-
  Add1 : Sum
  Add2 : Sum  Inputs=+-
  CT : Constant  Value=1.116e-5
  Fcn : Fcn  Expr=u(1)^2
  Fcn1 : Fcn  Expr=u(1)^2
  Jxx : Constant  Value=1.745e-2
  Jzz : Constant  Value=3.175e-2
  Product : Product
  Product1 : Product
  Product2 : Product  Inputs=3
  d : Constant  Value=0.225
  Out1 : Outport  VectorParamsAs1DForOutWhenUnconnected=off
  wires:
  Product2/1 -> Add1/1
  Fcn/1 -> Add2/2
  CT/1 -> Product2/3
  Jxx/1 -> Add/2
  Add1/1 -> 1/Jxx/1
  Fcn1/1 -> Add2/1
  Add2/1 -> Product2/1
  Product1/1 -> Add1/2
  Product/1 -> Product1/2
  d/1 -> Product2/2
  In4/1 -> Product/2
  Jzz/1 -> Add/1
  w1/1 -> Fcn/1
  Add/1 -> Product1/1
  1/Jxx/1 -> Out1/1
  w3/1 -> Fcn1/1
  In3/1 -> Product/1

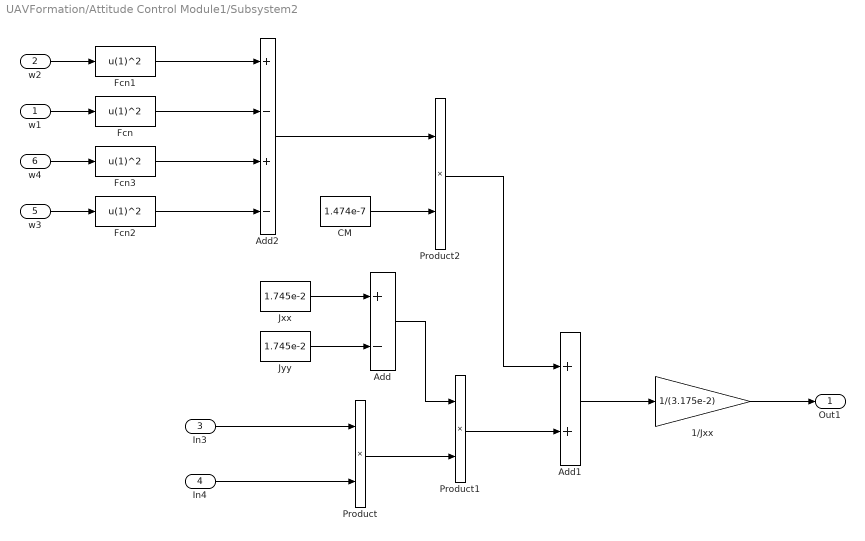
== system UAVFormation/Attitude Control Module1/Subsystem2 ==
  w1 : Inport
  w2 : Inport  Port=2
  In3 : Inport  Port=3
  In4 : Inport  Port=4
  w3 : Inport  Port=5
  w4 : Inport  Port=6
  1/Jxx : Gain  Gain=1/(3.175e-2)
  Add : Sum  Inputs=+-
  Add1 : Sum
  Add2 : Sum  Inputs=+-+-
  CM : Constant  Value=1.474e-7
  Fcn{,1..3} (4 alike) : Fcn  Expr=u(1)^2
  Jxx : Constant  Value=1.745e-2
  Jyy : Constant  Value=1.745e-2
  Product : Product
  Product1 : Product
  Product2 : Product
  Out1 : Outport  VectorParamsAs1DForOutWhenUnconnected=off
  wires:
  Product2/1 -> Add1/1
  CM/1 -> Product2/2
  Jyy/1 -> Add/2
  Add1/1 -> 1/Jxx/1
  Add2/1 -> Product2/1
  Product1/1 -> Add1/2
  Product/1 -> Product1/2
  In4/1 -> Product/2
  Jxx/1 -> Add/1
  Add/1 -> Product1/1
  1/Jxx/1 -> Out1/1
  In3/1 -> Product/1
  Fcn1/1 -> Add2/1
  Fcn/1 -> Add2/2
  Fcn3/1 -> Add2/3
  Fcn2/1 -> Add2/4
  w2/1 -> Fcn1/1
  w4/1 -> Fcn3/1
  w1/1 -> Fcn/1
  w3/1 -> Fcn2/1

== system UAVFormation/Attitude Control Module2/Subsystem ==
  w2 : Inport
  w4 : Inport  Port=2
  In3 : Inport  Port=3
  In4 : Inport  Port=4
  1/Jxx : Gain  Gain=1/(1.745e-2)
  Add : Sum  Inputs=+-
  Add1 : Sum
  Add2 : Sum  Inputs=+-
  CT : Constant  Value=1.116e-5
  Fcn : Fcn  Expr=u(1)^2
  Fcn1 : Fcn  Expr=u(1)^2
  Jyy : Constant  Value=1.745e-2
  "Jzz " : Constant  Value=3.175e-2
  Product : Product
  Product1 : Product
  Product2 : Product  Inputs=3
  d : Constant  Value=0.225
  Out1 : Outport  VectorParamsAs1DForOutWhenUnconnected=off
  wires:
  Product2/1 -> Add1/1
  Fcn/1 -> Add2/2
  CT/1 -> Product2/3
  "Jzz "/1 -> Add/2
  Add1/1 -> 1/Jxx/1
  Fcn1/1 -> Add2/1
  Add2/1 -> Product2/1
  Product1/1 -> Add1/2
  Product/1 -> Product1/2
  d/1 -> Product2/2
  In4/1 -> Product/2
  Jyy/1 -> Add/1
  w4/1 -> Fcn/1
  Add/1 -> Product1/1
  1/Jxx/1 -> Out1/1
  w2/1 -> Fcn1/1
  In3/1 -> Product/1

== system UAVFormation/Attitude Control Module2/Subsystem1 ==
  w3 : Inport
  w1 : Inport  Port=2
  In3 : Inport  Port=3
  In4 : Inport  Port=4
  1/Jxx : Gain  Gain=1/(1.745e-2)
  Add : Sum  Inputs=+-
  Add1 : Sum
  Add2 : Sum  Inputs=+-
  CT : Constant  Value=1.116e-5
  Fcn : Fcn  Expr=u(1)^2
  Fcn1 : Fcn  Expr=u(1)^2
  Jxx : Constant  Value=1.745e-2
  Jzz : Constant  Value=3.175e-2
  Product : Product
  Product1 : Product
  Product2 : Product  Inputs=3
  d : Constant  Value=0.225
  Out1 : Outport  VectorParamsAs1DForOutWhenUnconnected=off
  wires:
  Product2/1 -> Add1/1
  Fcn/1 -> Add2/2
  CT/1 -> Product2/3
  Jxx/1 -> Add/2
  Add1/1 -> 1/Jxx/1
  Fcn1/1 -> Add2/1
  Add2/1 -> Product2/1
  Product1/1 -> Add1/2
  Product/1 -> Product1/2
  d/1 -> Product2/2
  In4/1 -> Product/2
  Jzz/1 -> Add/1
  w1/1 -> Fcn/1
  Add/1 -> Product1/1
  1/Jxx/1 -> Out1/1
  w3/1 -> Fcn1/1
  In3/1 -> Product/1

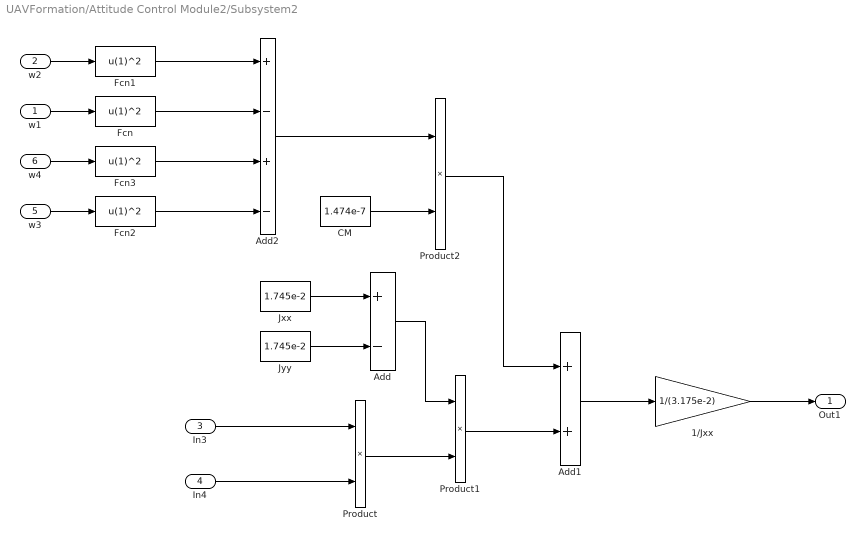
== system UAVFormation/Attitude Control Module2/Subsystem2 ==
  w1 : Inport
  w2 : Inport  Port=2
  In3 : Inport  Port=3
  In4 : Inport  Port=4
  w3 : Inport  Port=5
  w4 : Inport  Port=6
  1/Jxx : Gain  Gain=1/(3.175e-2)
  Add : Sum  Inputs=+-
  Add1 : Sum
  Add2 : Sum  Inputs=+-+-
  CM : Constant  Value=1.474e-7
  Fcn{,1..3} (4 alike) : Fcn  Expr=u(1)^2
  Jxx : Constant  Value=1.745e-2
  Jyy : Constant  Value=1.745e-2
  Product : Product
  Product1 : Product
  Product2 : Product
  Out1 : Outport  VectorParamsAs1DForOutWhenUnconnected=off
  wires:
  Product2/1 -> Add1/1
  CM/1 -> Product2/2
  Jyy/1 -> Add/2
  Add1/1 -> 1/Jxx/1
  Add2/1 -> Product2/1
  Product1/1 -> Add1/2
  Product/1 -> Product1/2
  In4/1 -> Product/2
  Jxx/1 -> Add/1
  Add/1 -> Product1/1
  1/Jxx/1 -> Out1/1
  In3/1 -> Product/1
  Fcn1/1 -> Add2/1
  Fcn/1 -> Add2/2
  Fcn3/1 -> Add2/3
  Fcn2/1 -> Add2/4
  w2/1 -> Fcn1/1
  w4/1 -> Fcn3/1
  w1/1 -> Fcn/1
  w3/1 -> Fcn2/1

== system UAVFormation/Attitude Control Module3/Subsystem ==
  w2 : Inport
  w4 : Inport  Port=2
  In3 : Inport  Port=3
  In4 : Inport  Port=4
  1/Jxx : Gain  Gain=1/(1.745e-2)
  Add : Sum  Inputs=+-
  Add1 : Sum
  Add2 : Sum  Inputs=+-
  CT : Constant  Value=1.116e-5
  Fcn : Fcn  Expr=u(1)^2
  Fcn1 : Fcn  Expr=u(1)^2
  Jyy : Constant  Value=1.745e-2
  "Jzz " : Constant  Value=3.175e-2
  Product : Product
  Product1 : Product
  Product2 : Product  Inputs=3
  d : Constant  Value=0.225
  Out1 : Outport  VectorParamsAs1DForOutWhenUnconnected=off
  wires:
  Product2/1 -> Add1/1
  Fcn/1 -> Add2/2
  CT/1 -> Product2/3
  "Jzz "/1 -> Add/2
  Add1/1 -> 1/Jxx/1
  Fcn1/1 -> Add2/1
  Add2/1 -> Product2/1
  Product1/1 -> Add1/2
  Product/1 -> Product1/2
  d/1 -> Product2/2
  In4/1 -> Product/2
  Jyy/1 -> Add/1
  w4/1 -> Fcn/1
  Add/1 -> Product1/1
  1/Jxx/1 -> Out1/1
  w2/1 -> Fcn1/1
  In3/1 -> Product/1

== system UAVFormation/Attitude Control Module3/Subsystem1 ==
  w3 : Inport
  w1 : Inport  Port=2
  In3 : Inport  Port=3
  In4 : Inport  Port=4
  1/Jxx : Gain  Gain=1/(1.745e-2)
  Add : Sum  Inputs=+-
  Add1 : Sum
  Add2 : Sum  Inputs=+-
  CT : Constant  Value=1.116e-5
  Fcn : Fcn  Expr=u(1)^2
  Fcn1 : Fcn  Expr=u(1)^2
  Jxx : Constant  Value=1.745e-2
  Jzz : Constant  Value=3.175e-2
  Product : Product
  Product1 : Product
  Product2 : Product  Inputs=3
  d : Constant  Value=0.225
  Out1 : Outport  VectorParamsAs1DForOutWhenUnconnected=off
  wires:
  Product2/1 -> Add1/1
  Fcn/1 -> Add2/2
  CT/1 -> Product2/3
  Jxx/1 -> Add/2
  Add1/1 -> 1/Jxx/1
  Fcn1/1 -> Add2/1
  Add2/1 -> Product2/1
  Product1/1 -> Add1/2
  Product/1 -> Product1/2
  d/1 -> Product2/2
  In4/1 -> Product/2
  Jzz/1 -> Add/1
  w1/1 -> Fcn/1
  Add/1 -> Product1/1
  1/Jxx/1 -> Out1/1
  w3/1 -> Fcn1/1
  In3/1 -> Product/1

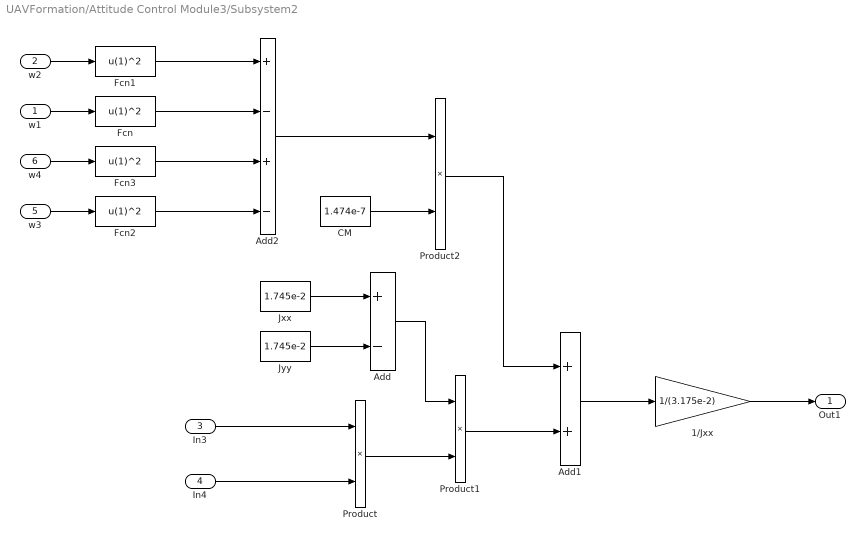
== system UAVFormation/Attitude Control Module3/Subsystem2 ==
  w1 : Inport
  w2 : Inport  Port=2
  In3 : Inport  Port=3
  In4 : Inport  Port=4
  w3 : Inport  Port=5
  w4 : Inport  Port=6
  1/Jxx : Gain  Gain=1/(3.175e-2)
  Add : Sum  Inputs=+-
  Add1 : Sum
  Add2 : Sum  Inputs=+-+-
  CM : Constant  Value=1.474e-7
  Fcn{,1..3} (4 alike) : Fcn  Expr=u(1)^2
  Jxx : Constant  Value=1.745e-2
  Jyy : Constant  Value=1.745e-2
  Product : Product
  Product1 : Product
  Product2 : Product
  Out1 : Outport  VectorParamsAs1DForOutWhenUnconnected=off
  wires:
  Product2/1 -> Add1/1
  CM/1 -> Product2/2
  Jyy/1 -> Add/2
  Add1/1 -> 1/Jxx/1
  Add2/1 -> Product2/1
  Product1/1 -> Add1/2
  Product/1 -> Product1/2
  In4/1 -> Product/2
  Jxx/1 -> Add/1
  Add/1 -> Product1/1
  1/Jxx/1 -> Out1/1
  In3/1 -> Product/1
  Fcn1/1 -> Add2/1
  Fcn/1 -> Add2/2
  Fcn3/1 -> Add2/3
  Fcn2/1 -> Add2/4
  w2/1 -> Fcn1/1
  w4/1 -> Fcn3/1
  w1/1 -> Fcn/1
  w3/1 -> Fcn2/1

== system UAVFormation/Attitude Control Module4/Subsystem ==
  w2 : Inport
  w4 : Inport  Port=2
  In3 : Inport  Port=3
  In4 : Inport  Port=4
  1/Jxx : Gain  Gain=1/(1.745e-2)
  Add : Sum  Inputs=+-
  Add1 : Sum
  Add2 : Sum  Inputs=+-
  CT : Constant  Value=1.116e-5
  Fcn : Fcn  Expr=u(1)^2
  Fcn1 : Fcn  Expr=u(1)^2
  Jyy : Constant  Value=1.745e-2
  "Jzz " : Constant  Value=3.175e-2
  Product : Product
  Product1 : Product
  Product2 : Product  Inputs=3
  d : Constant  Value=0.225
  Out1 : Outport  VectorParamsAs1DForOutWhenUnconnected=off
  wires:
  Product2/1 -> Add1/1
  Fcn/1 -> Add2/2
  CT/1 -> Product2/3
  "Jzz "/1 -> Add/2
  Add1/1 -> 1/Jxx/1
  Fcn1/1 -> Add2/1
  Add2/1 -> Product2/1
  Product1/1 -> Add1/2
  Product/1 -> Product1/2
  d/1 -> Product2/2
  In4/1 -> Product/2
  Jyy/1 -> Add/1
  w4/1 -> Fcn/1
  Add/1 -> Product1/1
  1/Jxx/1 -> Out1/1
  w2/1 -> Fcn1/1
  In3/1 -> Product/1

== system UAVFormation/Attitude Control Module4/Subsystem1 ==
  w3 : Inport
  w1 : Inport  Port=2
  In3 : Inport  Port=3
  In4 : Inport  Port=4
  1/Jxx : Gain  Gain=1/(1.745e-2)
  Add : Sum  Inputs=+-
  Add1 : Sum
  Add2 : Sum  Inputs=+-
  CT : Constant  Value=1.116e-5
  Fcn : Fcn  Expr=u(1)^2
  Fcn1 : Fcn  Expr=u(1)^2
  Jxx : Constant  Value=1.745e-2
  Jzz : Constant  Value=3.175e-2
  Product : Product
  Product1 : Product
  Product2 : Product  Inputs=3
  d : Constant  Value=0.225
  Out1 : Outport  VectorParamsAs1DForOutWhenUnconnected=off
  wires:
  Product2/1 -> Add1/1
  Fcn/1 -> Add2/2
  CT/1 -> Product2/3
  Jxx/1 -> Add/2
  Add1/1 -> 1/Jxx/1
  Fcn1/1 -> Add2/1
  Add2/1 -> Product2/1
  Product1/1 -> Add1/2
  Product/1 -> Product1/2
  d/1 -> Product2/2
  In4/1 -> Product/2
  Jzz/1 -> Add/1
  w1/1 -> Fcn/1
  Add/1 -> Product1/1
  1/Jxx/1 -> Out1/1
  w3/1 -> Fcn1/1
  In3/1 -> Product/1

== system UAVFormation/Attitude Control Module4/Subsystem2 ==
  w1 : Inport
  w2 : Inport  Port=2
  In3 : Inport  Port=3
  In4 : Inport  Port=4
  w3 : Inport  Port=5
  w4 : Inport  Port=6
  1/Jxx : Gain  Gain=1/(3.175e-2)
  Add : Sum  Inputs=+-
  Add1 : Sum
  Add2 : Sum  Inputs=+-+-
  CM : Constant  Value=1.474e-7
  Fcn{,1..3} (4 alike) : Fcn  Expr=u(1)^2
  Jxx : Constant  Value=1.745e-2
  Jyy : Constant  Value=1.745e-2
  Product : Product
  Product1 : Product
  Product2 : Product
  Out1 : Outport  VectorParamsAs1DForOutWhenUnconnected=off
  wires:
  Product2/1 -> Add1/1
  CM/1 -> Product2/2
  Jyy/1 -> Add/2
  Add1/1 -> 1/Jxx/1
  Add2/1 -> Product2/1
  Product1/1 -> Add1/2
  Product/1 -> Product1/2
  In4/1 -> Product/2
  Jxx/1 -> Add/1
  Add/1 -> Product1/1
  1/Jxx/1 -> Out1/1
  In3/1 -> Product/1
  Fcn1/1 -> Add2/1
  Fcn/1 -> Add2/2
  Fcn3/1 -> Add2/3
  Fcn2/1 -> Add2/4
  w2/1 -> Fcn1/1
  w4/1 -> Fcn3/1
  w1/1 -> Fcn/1
  w3/1 -> Fcn2/1

== matlab function UAVFormation/MATLAB Function6 ==
  data: u1 input; phi output; u2 input; u3 input; theta output; psai output
function [phi, theta, psai] = fcn(u1, u2, u3)

    phi = rem(u1,2*pi);
    theta = rem(u2,2*pi);
    psai = rem(u3,2*pi);
end

== matlab function UAVFormation/Position3 ==
  data: Ux input; U1 output; Uy input; Uz input; psaid input; m input; phid output; thetad output
function [U1,phid,thetad] = fcn(Ux,Uy,Uz,psaid,m)
    U1 = m*sqrt(Ux^2+Uy^2+(Uz+9.81)^2);
    phid = asin((Ux*sin(psaid)-Uy*cos(psaid))*m/U1);
%     thetad = asin((Ux*m-U1*sin(psaid)*sin(phid))/(U1*cos(psaid)*cos(phid)));
thetad=atan((Ux*cos(psaid)+Uy*sin(psaid))/(Uz+9.81));
end

== matlab function UAVFormation/MATLAB Function7 ==
  data: U1 input; w1 output; U2 input; U3 input; U4 input; w2 output; w3 output; w4 output
function [w1,w2,w3,w4] = fcn(U1,U2,U3,U4)
    CT = 1.116e-5; dCT = 0.225*CT;
    matrixA = [CT,CT,CT,CT;0,CT,0,-CT;-CT,0,CT,0;-dCT,dCT,-dCT,dCT];
    w_2 = inv(matrixA)*[U1,U2,U3,U4]';
    w1 = sqrt(abs(w_2(1))); w2 = sqrt(abs(w_2(2)));
    w3 = sqrt(abs(w_2(3))); w4 = sqrt(abs(w_2(4)));
end

== matlab function UAVFormation/MATLAB Function5 ==
  data: u1 input; phi output; u2 input; u3 input; theta output; psai output
function [phi, theta, psai] = fcn(u1, u2, u3)

    phi = rem(u1,2*pi);
    theta = rem(u2,2*pi);
    psai = rem(u3,2*pi);
end

== matlab function UAVFormation/MATLAB Function8 ==
  data: u1 input; phi output; u2 input; u3 input; theta output; psai output
function [phi, theta, psai] = fcn(u1, u2, u3)

    phi = rem(u1,2*pi);
    theta = rem(u2,2*pi);
    psai = rem(u3,2*pi);
end

== matlab function UAVFormation/Position4 ==
  data: Ux input; U1 output; Uy input; Uz input; psaid input; m input; phid output; thetad output
function [U1,phid,thetad] = fcn(Ux,Uy,Uz,psaid,m)
    U1 = m*sqrt(Ux^2+Uy^2+(Uz+9.81)^2);
    phid = asin((Ux*sin(psaid)-Uy*cos(psaid))*m/U1);
%     thetad = asin((Ux*m-U1*sin(psaid)*sin(phid))/(U1*cos(psaid)*cos(phid)));
thetad=atan((Ux*cos(psaid)+Uy*sin(psaid))/(Uz+9.81));
end

== matlab function UAVFormation/MATLAB Function2 ==
  data: U1 input; w1 output; U2 input; U3 input; U4 input; w2 output; w3 output; w4 output
function [w1,w2,w3,w4] = fcn(U1,U2,U3,U4)
    CT = 1.116e-5; dCT = 0.225*CT;
    matrixA = [CT,CT,CT,CT;0,CT,0,-CT;-CT,0,CT,0;-dCT,dCT,-dCT,dCT];
    w_2 = inv(matrixA)*[U1,U2,U3,U4]';
    w1 = sqrt(abs(w_2(1))); w2 = sqrt(abs(w_2(2)));
    w3 = sqrt(abs(w_2(3))); w4 = sqrt(abs(w_2(4)));
end

== matlab function UAVFormation/MATLAB Function1 ==
  data: U1 input; w1 output; U2 input; U3 input; U4 input; w2 output; w3 output; w4 output
function [w1,w2,w3,w4] = fcn(U1,U2,U3,U4)
    CT = 1.116e-5; dCT = 0.225*CT;
    matrixA = [CT,CT,CT,CT;0,CT,0,-CT;-CT,0,CT,0;-dCT,dCT,-dCT,dCT];
    w_2 = inv(matrixA)*[U1,U2,U3,U4]';
    w1 = sqrt(abs(w_2(1))); w2 = sqrt(abs(w_2(2)));
    w3 = sqrt(abs(w_2(3))); w4 = sqrt(abs(w_2(4)));
end

== matlab function UAVFormation/Position1 ==
  data: Ux input; U1 output; Uy input; Uz input; psaid input; m input; phid output; thetad output
function [U1,phid,thetad] = fcn(Ux,Uy,Uz,psaid,m)
    U1 = m*sqrt(Ux^2+Uy^2+(Uz+9.81)^2);
    phid = asin((Ux*sin(psaid)-Uy*cos(psaid))*m/U1);
%     thetad = asin((Ux*m-U1*sin(psaid)*sin(phid))/(U1*cos(psaid)*cos(phid)));
thetad=atan((Ux*cos(psaid)+Uy*sin(psaid))/(Uz+9.81));
end

== matlab function UAVFormation/MATLAB Function3 ==
  data: u1 input; phi output; u2 input; u3 input; theta output; psai output
function [phi, theta, psai] = fcn(u1, u2, u3)

    phi = rem(u1,2*pi);
    theta = rem(u2,2*pi);
    psai = rem(u3,2*pi);
end

== matlab function UAVFormation/Position2 ==
  data: Ux input; U1 output; Uy input; Uz input; psaid input; m input; phid output; thetad output
function [U1,phid,thetad] = fcn(Ux,Uy,Uz,psaid,m)
    U1 = m*sqrt(Ux^2+Uy^2+(Uz+9.81)^2);
    phid = asin((Ux*sin(psaid)-Uy*cos(psaid))*m/U1);
%     thetad = asin((Ux*m-U1*sin(psaid)*sin(phid))/(U1*cos(psaid)*cos(phid)));
thetad=atan((Ux*cos(psaid)+Uy*sin(psaid))/(Uz+9.81));
end
